simulink model "ZF_3"  (Simulink 7.7)
settings: Solver=VariableStepDiscrete  StartTime=0.0  StopTime=28  RelTol=1e-3
undefined symbols (not defined in the file or in its folder): get
libraries: dspsigops x2, commsink2 x1, simulink x1, dspsnks4 x1
settings Model: Creator=horacio  LastModifiedBy=horacio

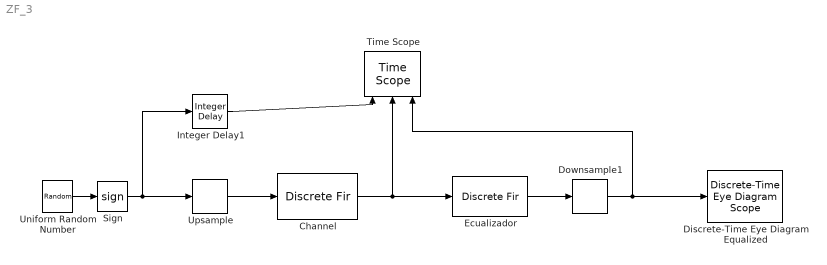
== system ZF_3 ==
  Channel : DiscreteFir  NumCoeffs=x
  Discrete-Time Eye Diagram Equalized : commsink2/Discrete-Time Eye Diagram Scope  Tag=EyeDiagram  SystemSampleTime=-1  sampPerSymb=8  offsetEye=0  symbPerTrace=4  numTraces=10  numNewFrames=10  LineStyles=-  LineColors=[0 0 0]  dupPoints=on  fading=on  render=on  AxisGrid=on  yMin=-4.48439305238087  yMax=4.25918206372825  inphaseLabel=In-phase Amplitude  quadratureLabel=Quadrature Amplitude  openScopeAtSimStart=on  dispDiagram=In-phase Only  FrameNumber=off  FigPos=get(0,'defaultfigureposition');  figTitle=Eye Diagram  block_type_=eye  numLinesMax=8
  Downsample1 : dspsigops/Downsample  N=2  phase=0  RateOptions=Allow multirate processing  smode=Allow multirate  fmode=Maintain input frame size  ic=0
  Ecualizador : DiscreteFir  NumCoeffs=[-2.2 4.9 -3 4.9 -2.2]
  Integer Delay1 : simulink/Discrete/Integer Delay  NumDelays=6  vinit=0.0  samptime=-1
  Sign : Signum
  Time Scope : dspsnks4/Time Scope  NumInputPorts=3
  Uniform Random Number : UniformRandomNumber  Seed=1  SampleTime=0.1
  Upsample : dspsigops/Upsample  N=2  phase=0  RateOptions=Allow multirate processing  ic=0  mode=Unused parameter value
  wires:
  Downsample1/1 -> Discrete-Time Eye Diagram Equalized/1, Time Scope/3
  Upsample/1 -> Channel/1
  Sign/1 -> Upsample/1, Integer Delay1/1
  Uniform Random Number/1 -> Sign/1
  Ecualizador/1 -> Downsample1/1
  Integer Delay1/1 -> Time Scope/1
  Channel/1 -> Ecualizador/1, Time Scope/2
